simulink model "ECE141_Project_1"  (R2019b)
settings: Solver=VariableStepAuto  StartTime=0.0  StopTime=140.0  RelTol=1e-9
settings Model: Creator=stephenchu  LastModifiedBy=stephenchu

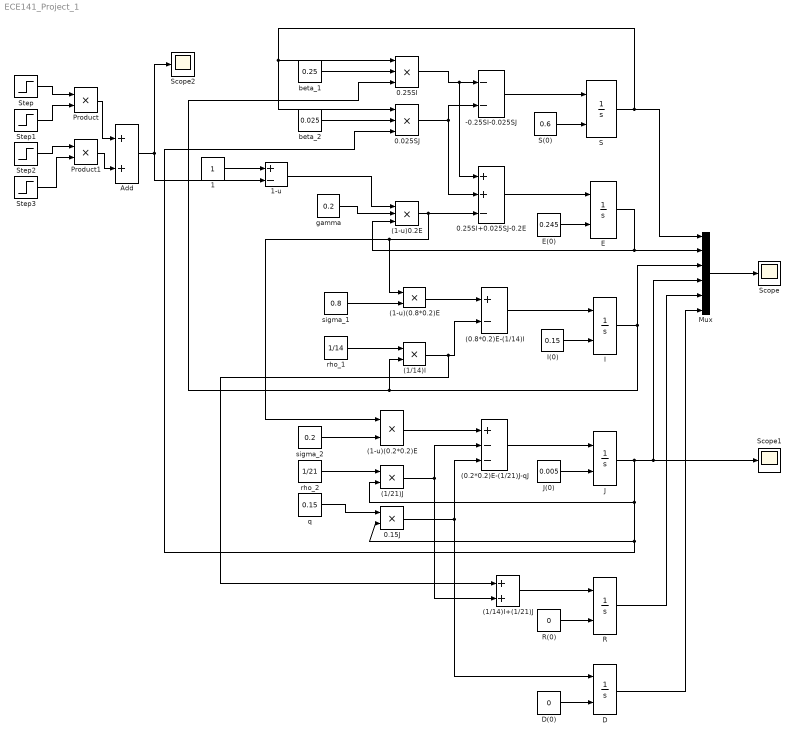
== system ECE141_Project_1 ==
  (0.2*0.2)E-(1/21)J-qJ : Sum  Inputs=+--
  (0.8*0.2)E-(1/14)I : Sum  Inputs=+-
  (1-u)(0.2*0.2)E : Product
  (1-u)(0.8*0.2)E : Product
  (1-u)0.2E : Product  Inputs=3
  (1/14)I : Product
  (1/14)I+(1/21)J : Sum
  (1/21)J : Product
  -0.25SI-0.025SJ : Sum  Inputs=--
  0.025SJ : Product  Inputs=3
  0.15J : Product
  0.25SI : Product  Inputs=3
  0.25SI+0.025SJ-0.2E : Sum  Inputs=++-
  "1 " : Constant
  1-u : Sum  Inputs=+-
  Add : Sum
  D : Integrator  InitialConditionSource=external
  D(0) : Constant  Value=0
  E : Integrator  InitialConditionSource=external
  E(0) : Constant  Value=0.245
  I : Integrator  InitialConditionSource=external
  I(0) : Constant  Value=0.15
  J : Integrator  InitialConditionSource=external
  J(0) : Constant  Value=0.005
  Mux : Mux  Inputs=6
  Product : Product
  Product1 : Product
  R : Integrator  InitialConditionSource=external
  R(0) : Constant  Value=0
  S : Integrator  InitialConditionSource=external
  S(0) : Constant  Value=0.6
  Scope : Scope
  Scope1 : Scope
  Scope2 : Scope
  Step : Step  Time=0  After=0.10  SampleTime=0
  Step1 : Step  Time=65  Before=1  After=0  SampleTime=0
  Step2 : Step  Time=0  After=0.70  SampleTime=0
  Step3 : Step  Time=90  Before=1  After=0  SampleTime=0
  beta_1 : Constant  Value=0.25
  beta_2 : Constant  Value=0.025
  gamma : Constant  Value=0.2
  q : Constant  Value=0.15
  rho_1 : Constant  Value=1/14
  rho_2 : Constant  Value=1/21
  sigma_1 : Constant  Value=0.8
  sigma_2 : Constant  Value=0.2
  wires:
  -0.25SI-0.025SJ/1 -> S/1
  S/1 -> Mux/1, 0.25SI/1, 0.025SJ/1
  beta_1/1 -> 0.25SI/2
  beta_2/1 -> 0.025SJ/2
  0.25SI/1 -> -0.25SI-0.025SJ/1, 0.25SI+0.025SJ-0.2E/1
  0.025SJ/1 -> 0.25SI+0.025SJ-0.2E/2, -0.25SI-0.025SJ/2
  0.25SI+0.025SJ-0.2E/1 -> E/1
  (1-u)0.2E/1 -> (1-u)(0.8*0.2)E/1, (1-u)(0.2*0.2)E/1, 0.25SI+0.025SJ-0.2E/3
  E/1 -> Mux/2, (1-u)0.2E/3
  gamma/1 -> (1-u)0.2E/2
  sigma_1/1 -> (1-u)(0.8*0.2)E/2
  (1-u)(0.8*0.2)E/1 -> (0.8*0.2)E-(1/14)I/1
  rho_1/1 -> (1/14)I/1
  I/1 -> Mux/3, 0.25SI/3, (1/14)I/2
  (1/14)I/1 -> (1/14)I+(1/21)J/1, (0.8*0.2)E-(1/14)I/2
  (0.8*0.2)E-(1/14)I/1 -> I/1
  sigma_2/1 -> (1-u)(0.2*0.2)E/2
  (1-u)(0.2*0.2)E/1 -> (0.2*0.2)E-(1/21)J-qJ/1
  (0.2*0.2)E-(1/21)J-qJ/1 -> J/1
  J/1 -> Scope1/1, Mux/4, 0.025SJ/3, 0.15J/2, (1/21)J/2
  rho_2/1 -> (1/21)J/1
  (1/21)J/1 -> (1/14)I+(1/21)J/2, (0.2*0.2)E-(1/21)J-qJ/2
  q/1 -> 0.15J/1
  0.15J/1 -> D/1, (0.2*0.2)E-(1/21)J-qJ/3
  (1/14)I+(1/21)J/1 -> R/1
  S(0)/1 -> S/2
  E(0)/1 -> E/2
  I(0)/1 -> I/2
  J(0)/1 -> J/2
  R(0)/1 -> R/2
  D(0)/1 -> D/2
  D/1 -> Mux/6
  R/1 -> Mux/5
  Mux/1 -> Scope/1
  Step/1 -> Product/1
  Step1/1 -> Product/2
  Step2/1 -> Product1/1
  Step3/1 -> Product1/2
  Product/1 -> Add/1
  Product1/1 -> Add/2
  Add/1 -> Scope2/1, 1-u/2
  "1 "/1 -> 1-u/1
  1-u/1 -> (1-u)0.2E/1
